simulink model "high_gain_observers"  (R2017a)
settings: Solver=VariableStepAuto  StartTime=0.0  StopTime=10  RelTol=1e-3
PreLoadFcn:
  | Mode = 1;
  | SFB = Simulink.Variant('Mode == 1');
  | OFB = Simulink.Variant('Mode == 2');
libraries: simulink x1
settings Model: Creator=29921  LastModifiedBy=29921

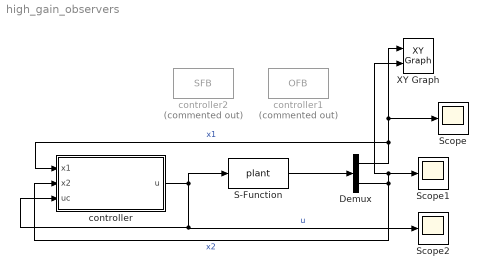
== system high_gain_observers ==
  Demux : Demux  Outputs=2
  S-Function : S-Function  FunctionName=plant  SFunctionDeploymentMode=off  EnableBusSupport=off
  Scope : Scope
  Scope1 : Scope
  Scope2 : Scope
  XY Graph : simulink/Sinks/XY Graph  xmin=-3  xmax=3  ymin=-2  ymax=2  st=-1
  controller : Subsystem  Variant=on
  controller1 : S-Function  Commented=on  FunctionName=OFB  SFunctionDeploymentMode=off  EnableBusSupport=off
  controller2 : S-Function  Commented=on  FunctionName=SFB  SFunctionDeploymentMode=off  EnableBusSupport=off
  wires:
  S-Function/1 -> Demux/1
  Demux/1 -> controller/1(x1), XY Graph/1, Scope/1  "x1"
  Demux/2 -> controller/2(x2), Scope1/1, XY Graph/2  "x2"
  controller/1(u) -> S-Function/1, controller/3(uc), Scope2/1  "u"

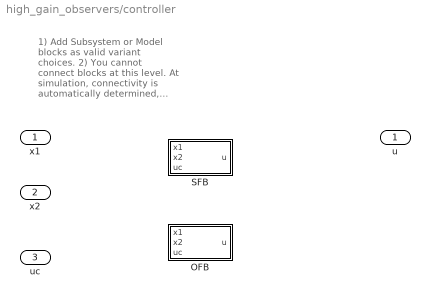
== system high_gain_observers/controller ==
  note: 1) Add Subsystem or Model blocks as valid variant choices.
      | 2) You cannot connect blocks at this level. At simulation, connectivity is automatically
      | determined, based on the active variant and port name matching.
  x1 : Inport
  x2 : Inport  Port=2
  uc : Inport  Port=3
  OFB : Subsystem  VariantControl=OFB
  SFB : Subsystem  VariantControl=SFB
  u : Outport

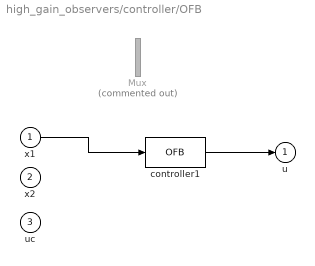
== system high_gain_observers/controller/OFB ==
  x1 : Inport
  x2 : Inport  Port=2
  uc : Inport  Port=3
  Mux : Mux  Commented=on  Inputs=2
  controller1 : S-Function  FunctionName=OFB  SFunctionDeploymentMode=off  EnableBusSupport=off
  u : Outport
  wires:
  controller1/1 -> u/1
  x1/1 -> controller1/1

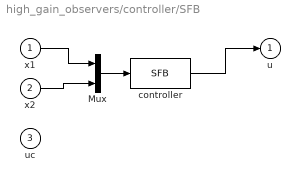
== system high_gain_observers/controller/SFB ==
  x1 : Inport
  x2 : Inport  Port=2
  uc : Inport  Port=3
  Mux : Mux  Inputs=2
  controller : S-Function  FunctionName=SFB  SFunctionDeploymentMode=off  EnableBusSupport=off
  u : Outport
  wires:
  x1/1 -> Mux/1
  x2/1 -> Mux/2
  Mux/1 -> controller/1
  controller/1 -> u/1
